simulink model "FullSystem"  (R2014a)
settings: Solver=ode45  StartTime=0.0  StopTime=.04  RelTol=1e-3
undefined symbols (not defined in the file): i
libraries: dspsigops x14, dspmtrx3 x7, dspsrcs4 x7
settings Model: Creator=Dolby  LastModifiedBy=100442260
settings DebuggingCC: UnderspecifiedInitializationDetection=Classic  StateNameClashWarn=warning

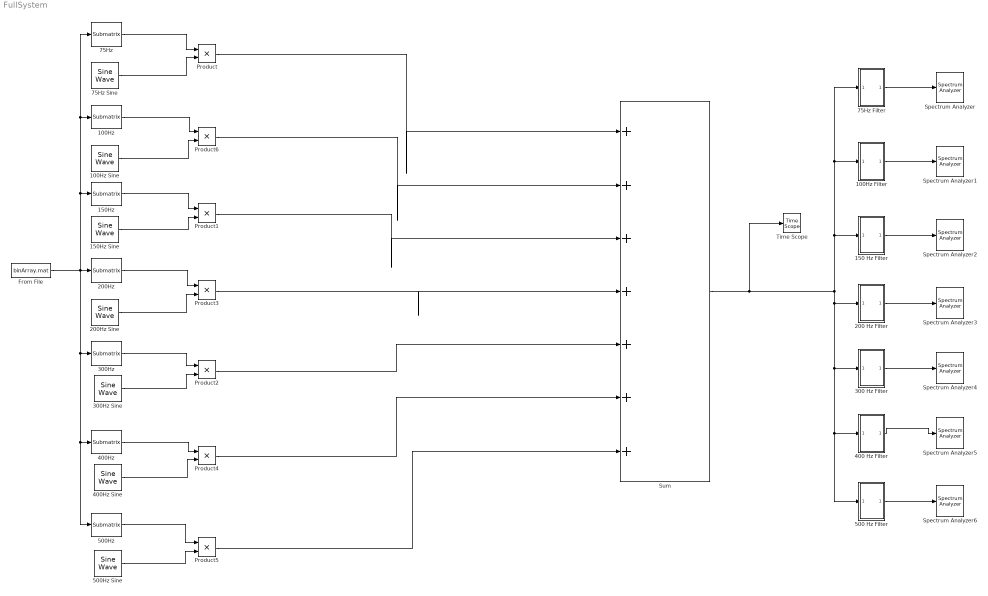
== system FullSystem ==
  100Hz : dspmtrx3/Submatrix  RowSpan=One row  RowStartMode=Index  RowStartIndex=2  RowEndMode=Last  RowEndIndex=1  ColSpan=Range of columns  ColStartMode=First  ColStartIndex=1  ColEndMode=Last  ColEndIndex=1
  100Hz Filter : Subsystem
  100Hz Sine : dspsrcs4/Sine Wave  Amplitude=1 + rand()  Frequency=100  Phase=0  SampleMode=Discrete  OutComplex=Real  CompMethod=Trigonometric fcn  TableSize=Speed  SampleTime=1/8000  SamplesPerFrame=1  ResetState=Restart at time zero  dataType=double  wordLen=16  udDataType=sfix(16)  fracBitsMode=Best precision  numFracBits=15  OutDataTypeStr=double  LastOutDataTypeStr=double
  150 Hz Filter : Subsystem
  150Hz : dspmtrx3/Submatrix  RowSpan=One row  RowStartMode=Index  RowStartIndex=3  RowEndMode=Last  RowEndIndex=1  ColSpan=Range of columns  ColStartMode=First  ColStartIndex=1  ColEndMode=Last  ColEndIndex=1
  150Hz Sine : dspsrcs4/Sine Wave  Amplitude=1 + rand()  Frequency=150  Phase=0  SampleMode=Discrete  OutComplex=Real  CompMethod=Trigonometric fcn  TableSize=Speed  SampleTime=1/8000  SamplesPerFrame=1  ResetState=Restart at time zero  dataType=double  wordLen=16  udDataType=sfix(16)  fracBitsMode=Best precision  numFracBits=15  OutDataTypeStr=double  LastOutDataTypeStr=double
  200 Hz Filter : Subsystem
  200Hz : dspmtrx3/Submatrix  RowSpan=One row  RowStartMode=Index  RowStartIndex=4  RowEndMode=Last  RowEndIndex=1  ColSpan=Range of columns  ColStartMode=First  ColStartIndex=1  ColEndMode=Last  ColEndIndex=1
  200Hz Sine : dspsrcs4/Sine Wave  Amplitude=1 + rand()  Frequency=200  Phase=0  SampleMode=Discrete  OutComplex=Real  CompMethod=Trigonometric fcn  TableSize=Speed  SampleTime=1/8000  SamplesPerFrame=1  ResetState=Restart at time zero  dataType=double  wordLen=16  udDataType=sfix(16)  fracBitsMode=Best precision  numFracBits=15  OutDataTypeStr=double  LastOutDataTypeStr=double
  "300 Hz Filter " : Subsystem
  300Hz : dspmtrx3/Submatrix  RowSpan=One row  RowStartMode=Index  RowStartIndex=5  RowEndMode=Last  RowEndIndex=1  ColSpan=Range of columns  ColStartMode=First  ColStartIndex=1  ColEndMode=Last  ColEndIndex=1
  300Hz Sine : dspsrcs4/Sine Wave  Amplitude=1 + rand()  Frequency=300  Phase=0  SampleMode=Discrete  OutComplex=Real  CompMethod=Trigonometric fcn  TableSize=Speed  SampleTime=1/8000  SamplesPerFrame=1  ResetState=Restart at time zero  dataType=double  wordLen=16  udDataType=sfix(16)  fracBitsMode=Best precision  numFracBits=15  OutDataTypeStr=double  LastOutDataTypeStr=double
  400 Hz Filter : Subsystem
  400Hz : dspmtrx3/Submatrix  RowSpan=One row  RowStartMode=Index  RowStartIndex=6  RowEndMode=Last  RowEndIndex=1  ColSpan=Range of columns  ColStartMode=First  ColStartIndex=1  ColEndMode=Last  ColEndIndex=1
  400Hz Sine : dspsrcs4/Sine Wave  Amplitude=1 + rand()  Frequency=200  Phase=0  SampleMode=Discrete  OutComplex=Real  CompMethod=Trigonometric fcn  TableSize=Speed  SampleTime=1/8000  SamplesPerFrame=1  ResetState=Restart at time zero  dataType=double  wordLen=16  udDataType=sfix(16)  fracBitsMode=Best precision  numFracBits=15  OutDataTypeStr=double  LastOutDataTypeStr=double
  500 Hz Filter : Subsystem
  500Hz : dspmtrx3/Submatrix  RowSpan=One row  RowStartMode=Last  RowStartIndex=1  RowEndMode=Last  RowEndIndex=1  ColSpan=Range of columns  ColStartMode=First  ColStartIndex=1  ColEndMode=Last  ColEndIndex=1
  500Hz Sine : dspsrcs4/Sine Wave  Amplitude=1 + rand()  Frequency=500  Phase=0  SampleMode=Discrete  OutComplex=Real  CompMethod=Trigonometric fcn  TableSize=Speed  SampleTime=1/8000  SamplesPerFrame=1  ResetState=Restart at time zero  dataType=double  wordLen=16  udDataType=sfix(16)  fracBitsMode=Best precision  numFracBits=15  OutDataTypeStr=double  LastOutDataTypeStr=double
  75Hz : dspmtrx3/Submatrix  RowSpan=One row  RowStartMode=First  RowStartIndex=1  RowEndMode=Last  RowEndIndex=1  ColSpan=Range of columns  ColStartMode=First  ColStartIndex=1  ColEndMode=Last  ColEndIndex=1
  75Hz Filter : Subsystem
  75Hz Sine : dspsrcs4/Sine Wave  Amplitude=1 + rand()  Frequency=75  Phase=0  SampleMode=Discrete  OutComplex=Real  CompMethod=Trigonometric fcn  TableSize=Speed  SampleTime=1/8000  SamplesPerFrame=1  ResetState=Restart at time zero  dataType=double  wordLen=16  udDataType=sfix(16)  fracBitsMode=Best precision  numFracBits=15  OutDataTypeStr=double  LastOutDataTypeStr=double
  From File : FromFile  FileName=binArray.mat  SampleTime=0  ExtrapolationBeforeFirstDataPoint=Ground value  InterpolationWithinTimeRange=Zero order hold  ExtrapolationAfterLastDataPoint=Ground value
  Product{,1..6} (7 alike) : Product
  Spectrum Analyzer{,1..6} (7 alike) : SpectrumAnalyzer
  Sum : Sum  Inputs=|+++++++
  Time Scope : TimeScope  DefaultConfigurationName=spbscopes.TimeScopeBlockCfg
  wires:
  From File/1 -> 100Hz/1, 75Hz/1, 150Hz/1, 500Hz/1, 400Hz/1, 300Hz/1, 200Hz/1
  150Hz/1 -> Product1/1
  150Hz Sine/1 -> Product1/2
  200Hz/1 -> Product3/1
  100Hz Sine/1 -> Product6/2
  100Hz/1 -> Product6/1
  300Hz/1 -> Product2/1
  75Hz/1 -> Product/1
  400Hz/1 -> Product4/1
  500Hz/1 -> Product5/1
  Product/1 -> Sum/1
  Product6/1 -> Sum/2
  Product1/1 -> Sum/3
  Product3/1 -> Sum/4
  Product2/1 -> Sum/5
  Product4/1 -> Sum/6
  Product5/1 -> Sum/7
  Sum/1 -> Time Scope/1, 150 Hz Filter/1(In1), 75Hz Filter/1(In1), 100Hz Filter/1(In1), 500 Hz Filter/1(In1), 400 Hz Filter/1(In1), "300 Hz Filter "/1(In1), 200 Hz Filter/1(In1)
  75Hz Sine/1 -> Product/2
  200Hz Sine/1 -> Product3/2
  300Hz Sine/1 -> Product2/2
  400Hz Sine/1 -> Product4/2
  500Hz Sine/1 -> Product5/2
  75Hz Filter/1(Out1) -> Spectrum Analyzer/1
  100Hz Filter/1(Out1) -> Spectrum Analyzer1/1
  150 Hz Filter/1(Out1) -> Spectrum Analyzer2/1
  200 Hz Filter/1(Out1) -> Spectrum Analyzer3/1
  "300 Hz Filter "/1(Out1) -> Spectrum Analyzer4/1
  400 Hz Filter/1(Out1) -> Spectrum Analyzer5/1
  500 Hz Filter/1(Out1) -> Spectrum Analyzer6/1

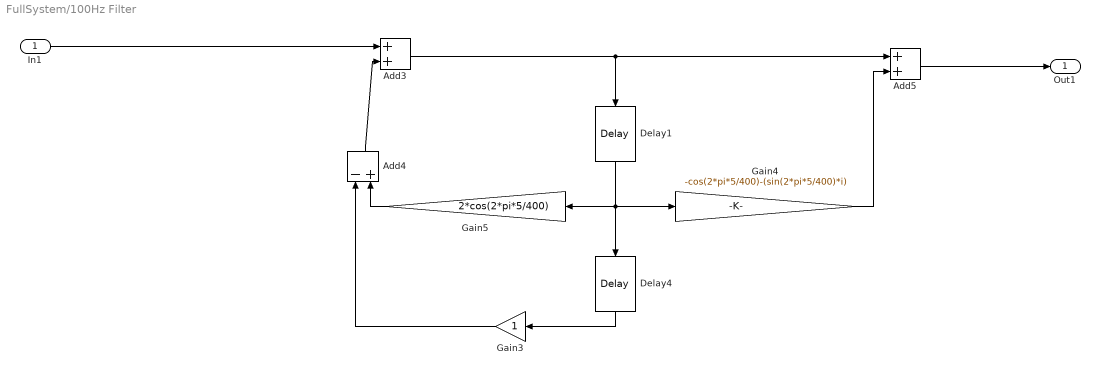
== system FullSystem/100Hz Filter ==
  In1 : Inport
  Add3 : Sum
  Add4 : Sum  Inputs=-+
  Add5 : Sum
  Delay1 : dspsigops/Delay  dly_unit=Samples  delay=1  ic_detail=off  dif_ic_for_ch=off  dif_ic_for_dly=off  ic=0  reset_popup=None
  Delay4 : dspsigops/Delay  dly_unit=Samples  delay=1  ic_detail=off  dif_ic_for_ch=off  dif_ic_for_dly=off  ic=0  reset_popup=None
  Gain3 : Gain
  Gain4 : Gain  Gain=-cos(2*pi*5/400)-(sin(2*pi*5/400)*i)
  Gain5 : Gain  Gain=2*cos(2*pi*5/400)
  Out1 : Outport
  wires:
  In1/1 -> Add3/1
  Add4/1 -> Add3/2
  Gain3/1 -> Add4/1
  Add3/1 -> Add5/1, Delay1/1
  Add5/1 -> Out1/1
  Gain5/1 -> Add4/2
  Gain4/1 -> Add5/2
  Delay4/1 -> Gain3/1
  Delay1/1 -> Gain4/1, Gain5/1, Delay4/1

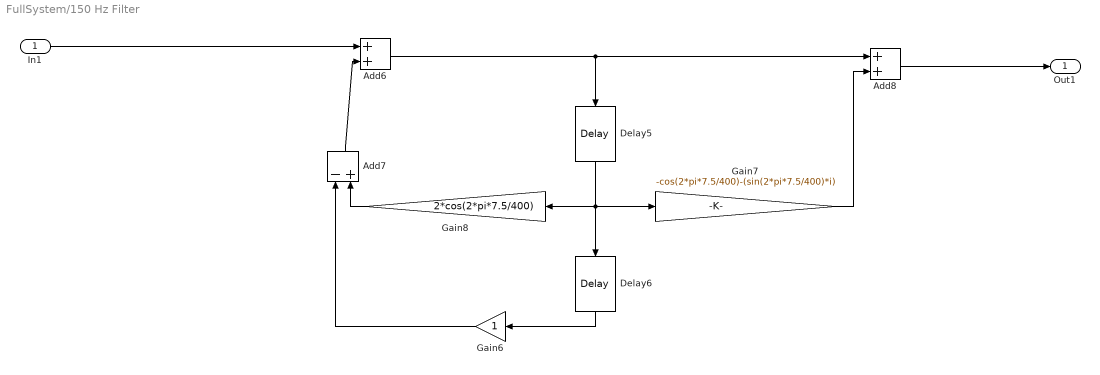
== system FullSystem/150 Hz Filter ==
  In1 : Inport
  Add6 : Sum
  Add7 : Sum  Inputs=-+
  Add8 : Sum
  Delay5 : dspsigops/Delay  dly_unit=Samples  delay=1  ic_detail=off  dif_ic_for_ch=off  dif_ic_for_dly=off  ic=0  reset_popup=None
  Delay6 : dspsigops/Delay  dly_unit=Samples  delay=1  ic_detail=off  dif_ic_for_ch=off  dif_ic_for_dly=off  ic=0  reset_popup=None
  Gain6 : Gain
  Gain7 : Gain  Gain=-cos(2*pi*7.5/400)-(sin(2*pi*7.5/400)*i)
  Gain8 : Gain  Gain=2*cos(2*pi*7.5/400)
  Out1 : Outport
  wires:
  In1/1 -> Add6/1
  Gain7/1 -> Add8/2
  Add8/1 -> Out1/1
  Delay5/1 -> Gain7/1, Gain8/1, Delay6/1
  Gain8/1 -> Add7/2
  Add6/1 -> Add8/1, Delay5/1
  Add7/1 -> Add6/2
  Delay6/1 -> Gain6/1
  Gain6/1 -> Add7/1

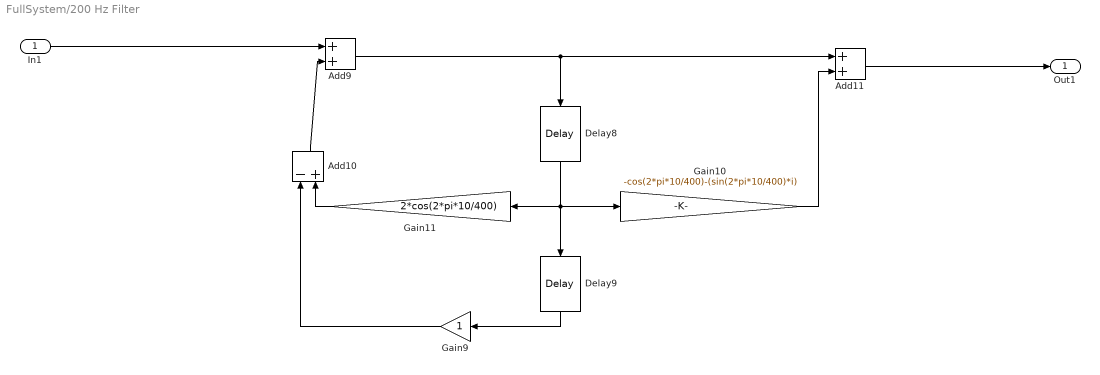
== system FullSystem/200 Hz Filter ==
  In1 : Inport
  Add10 : Sum  Inputs=-+
  Add11 : Sum
  Add9 : Sum
  Delay8 : dspsigops/Delay  dly_unit=Samples  delay=1  ic_detail=off  dif_ic_for_ch=off  dif_ic_for_dly=off  ic=0  reset_popup=None
  Delay9 : dspsigops/Delay  dly_unit=Samples  delay=1  ic_detail=off  dif_ic_for_ch=off  dif_ic_for_dly=off  ic=0  reset_popup=None
  Gain10 : Gain  Gain=-cos(2*pi*10/400)-(sin(2*pi*10/400)*i)
  Gain11 : Gain  Gain=2*cos(2*pi*10/400)
  Gain9 : Gain
  Out1 : Outport
  wires:
  Gain10/1 -> Add11/2
  Delay8/1 -> Gain10/1, Gain11/1, Delay9/1
  Gain9/1 -> Add10/1
  Add10/1 -> Add9/2
  Delay9/1 -> Gain9/1
  Add11/1 -> Out1/1
  Add9/1 -> Add11/1, Delay8/1
  Gain11/1 -> Add10/2
  In1/1 -> Add9/1

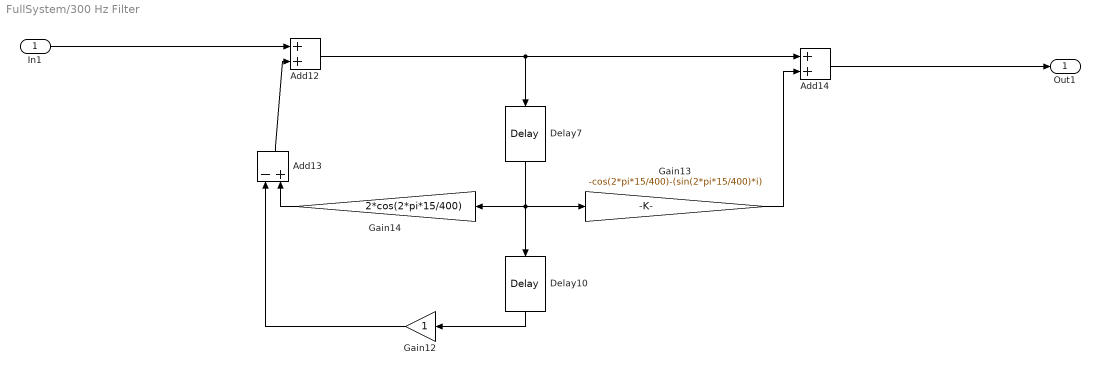
== system FullSystem/300 Hz Filter  ==
  In1 : Inport
  Add12 : Sum
  Add13 : Sum  Inputs=-+
  Add14 : Sum
  Delay10 : dspsigops/Delay  dly_unit=Samples  delay=1  ic_detail=off  dif_ic_for_ch=off  dif_ic_for_dly=off  ic=0  reset_popup=None
  Delay7 : dspsigops/Delay  dly_unit=Frames  delay=1  ic_detail=off  dif_ic_for_ch=off  dif_ic_for_dly=off  ic=0  reset_popup=None
  Gain12 : Gain
  Gain13 : Gain  Gain=-cos(2*pi*15/400)-(sin(2*pi*15/400)*i)
  Gain14 : Gain  Gain=2*cos(2*pi*15/400)
  Out1 : Outport
  wires:
  Add14/1 -> Out1/1
  Add12/1 -> Add14/1, Delay7/1
  Gain12/1 -> Add13/1
  Delay7/1 -> Gain13/1, Gain14/1, Delay10/1
  Add13/1 -> Add12/2
  Gain13/1 -> Add14/2
  Delay10/1 -> Gain12/1
  Gain14/1 -> Add13/2
  In1/1 -> Add12/1

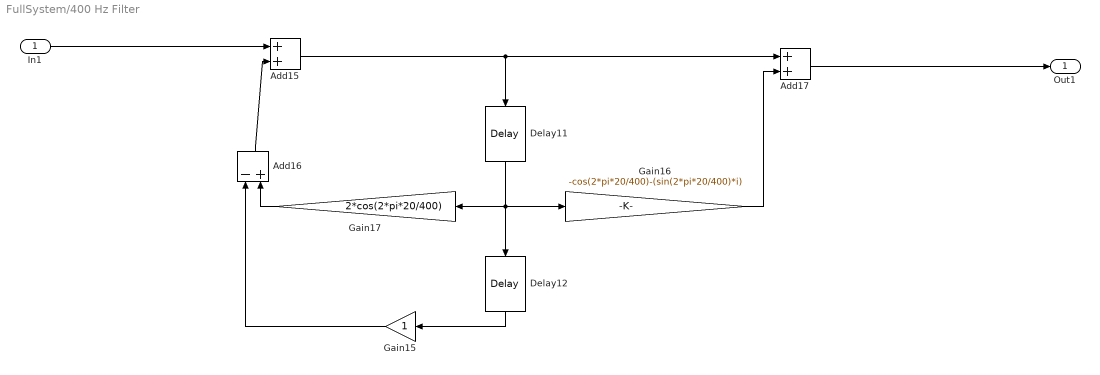
== system FullSystem/400 Hz Filter ==
  In1 : Inport
  Add15 : Sum
  Add16 : Sum  Inputs=-+
  Add17 : Sum
  Delay11 : dspsigops/Delay  dly_unit=Samples  delay=1  ic_detail=off  dif_ic_for_ch=off  dif_ic_for_dly=off  ic=0  reset_popup=None
  Delay12 : dspsigops/Delay  dly_unit=Samples  delay=1  ic_detail=off  dif_ic_for_ch=off  dif_ic_for_dly=off  ic=0  reset_popup=None
  Gain15 : Gain
  Gain16 : Gain  Gain=-cos(2*pi*20/400)-(sin(2*pi*20/400)*i)
  Gain17 : Gain  Gain=2*cos(2*pi*20/400)
  Out1 : Outport
  wires:
  Gain17/1 -> Add16/2
  Add16/1 -> Add15/2
  Add15/1 -> Add17/1, Delay11/1
  Gain15/1 -> Add16/1
  Delay11/1 -> Gain16/1, Gain17/1, Delay12/1
  Gain16/1 -> Add17/2
  Add17/1 -> Out1/1
  Delay12/1 -> Gain15/1
  In1/1 -> Add15/1

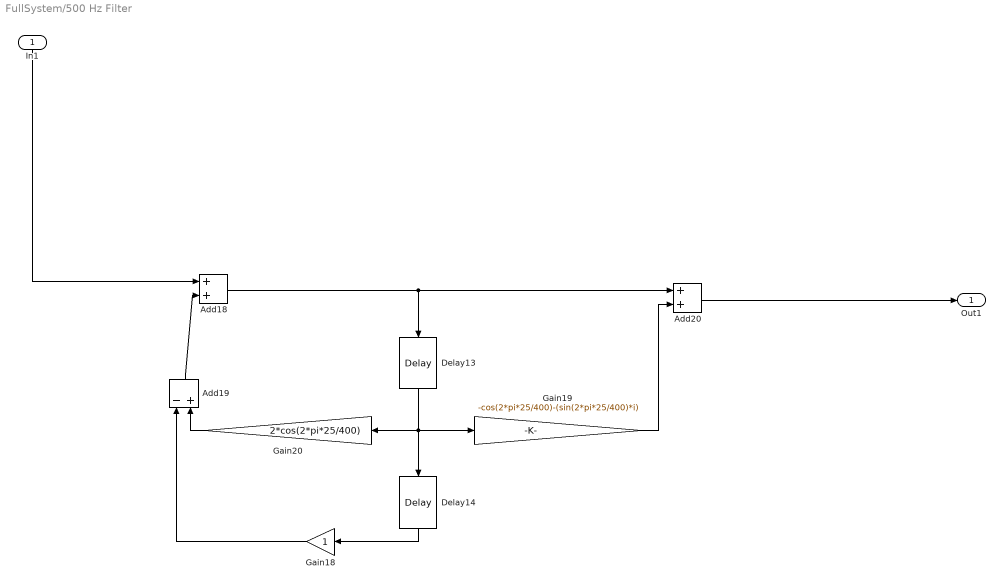
== system FullSystem/500 Hz Filter ==
  In1 : Inport
  Add18 : Sum
  Add19 : Sum  Inputs=-+
  Add20 : Sum
  Delay13 : dspsigops/Delay  dly_unit=Samples  delay=1  ic_detail=off  dif_ic_for_ch=off  dif_ic_for_dly=off  ic=0  reset_popup=None
  Delay14 : dspsigops/Delay  dly_unit=Samples  delay=1  ic_detail=off  dif_ic_for_ch=off  dif_ic_for_dly=off  ic=0  reset_popup=None
  Gain18 : Gain
  Gain19 : Gain  Gain=-cos(2*pi*25/400)-(sin(2*pi*25/400)*i)
  Gain20 : Gain  Gain=2*cos(2*pi*25/400)
  Out1 : Outport
  wires:
  Delay13/1 -> Gain19/1, Gain20/1, Delay14/1
  Add19/1 -> Add18/2
  Add18/1 -> Add20/1, Delay13/1
  Gain18/1 -> Add19/1
  Delay14/1 -> Gain18/1
  Add20/1 -> Out1/1
  Gain19/1 -> Add20/2
  Gain20/1 -> Add19/2
  In1/1 -> Add18/1

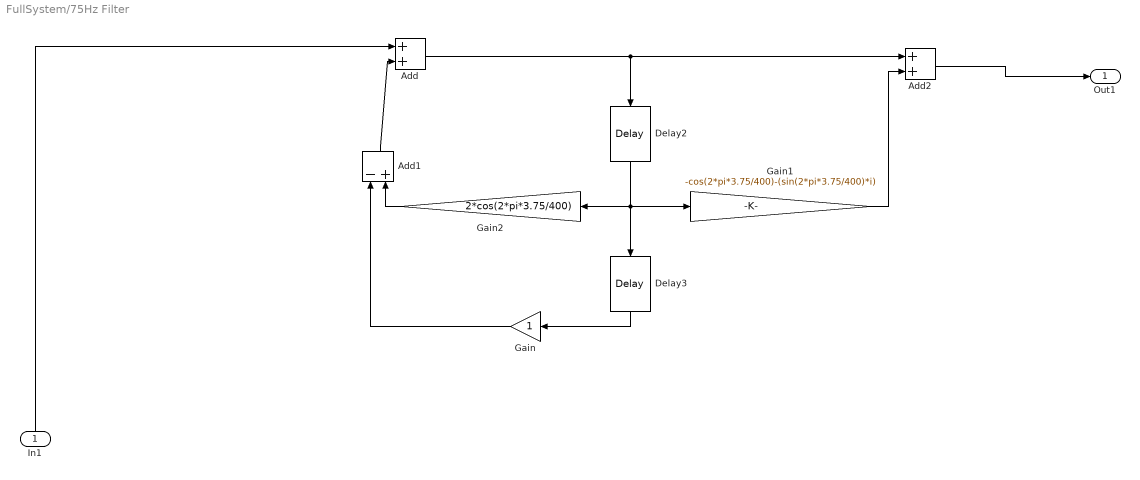
== system FullSystem/75Hz Filter ==
  In1 : Inport
  Add : Sum
  Add1 : Sum  Inputs=-+
  Add2 : Sum
  Delay2 : dspsigops/Delay  dly_unit=Samples  delay=1  ic_detail=off  dif_ic_for_ch=off  dif_ic_for_dly=off  ic=0  reset_popup=None
  Delay3 : dspsigops/Delay  InputProcessing=Columns as channels (frame based)  dly_unit=Frames  delay=1  ic_detail=off  dif_ic_for_ch=off  dif_ic_for_dly=off  ic=0  reset_popup=None
  Gain : Gain
  Gain1 : Gain  Gain=-cos(2*pi*3.75/400)-(sin(2*pi*3.75/400)*i)
  Gain2 : Gain  Gain=2*cos(2*pi*3.75/400)
  Out1 : Outport
  wires:
  In1/1 -> Add/1
  Add2/1 -> Out1/1
  Gain/1 -> Add1/1
  Gain2/1 -> Add1/2
  Gain1/1 -> Add2/2
  Add1/1 -> Add/2
  Add/1 -> Add2/1, Delay2/1
  Delay3/1 -> Gain/1
  Delay2/1 -> Gain1/1, Gain2/1, Delay3/1
